simulink model "practice"  (R2017a)
settings: Solver=FixedStepAuto  StartTime=0.0  StopTime=40000  FixedStep=1  RelTol=1e-3
settings Model: Creator=zhiangz  LastModifiedBy=zhiangz

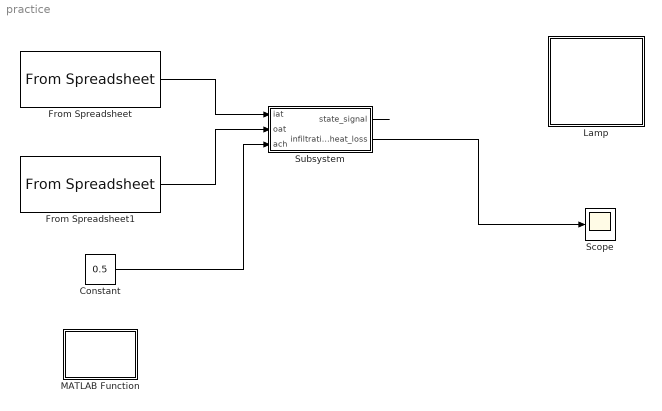
== system practice ==
  Constant : Constant  Value=0.5
  From Spreadsheet : FromSpreadsheet  FileName=indoor_air_temperature.csv  SheetName=indoor_air_temperature  SampleTime=-1
  From Spreadsheet1 : FromSpreadsheet  FileName=outdoor_air_temperature.csv  SheetName=outdoor_air_temperature  SampleTime=-1
  Lamp : Subsystem  DialogController=hmiCreateDDGDialog  IsWebBlock=on  mask(MWDashboardBlock){webBlockId=c2a7fa99-169d-49c1-9f26-a671b7992dc5, webBlockType=lamp, ShowInLibBrowser=on, ShowInitialText=on, HMISrcModelName=practice}
      mask prompts: webBlockType "WebBlock Type"; HMISrcModelName "Source Model"
      mask help: SimulinkHMI:dialogs:LampDialogDesc
      mask Help: helpview([docroot '/mapfiles/simulink.map'], 'hmi_lamp')
      mask Display:
      | if strcmp(get_param(bdroot(gcb),'BlockDiagramType'), 'library')
      |     image([(matlabroot) '/toolbox/simulink/hmi/icons/Lamp.png']);
      | end
  MATLAB Function : MATLAB Function  TreatAsAtomicUnit=on
  Scope : Scope
  Subsystem : Subsystem
  wires:
  From Spreadsheet/1 -> Subsystem/1(iat)
  From Spreadsheet1/1 -> Subsystem/2(oat)
  Subsystem/1(state_signal) -> ?
  Constant/1 -> Subsystem/3(ach)
  Subsystem/2(infiltration_heat_loss) -> Scope/1

== system practice/Lamp ==

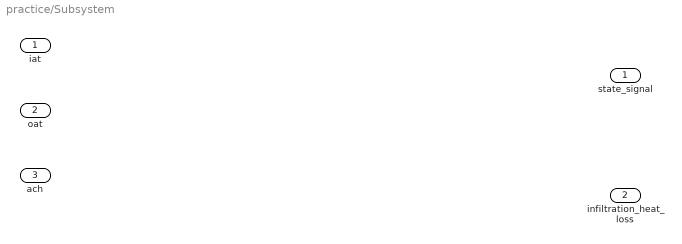
== system practice/Subsystem ==
  iat : Inport
  oat : Inport  Port=2
  ach : Inport  Port=3
  state_signal : Outport
  infiltration_heat_loss : Outport  Port=2

== matlab function practice/MATLAB Function ==
function fcn
pause(0.001);
